simulink subsystem "Encoder_SubSystem"  (R2020b)
settings: Solver=VariableStepAuto  StartTime=0.0  StopTime=10.0  RelTol=1e-3
undefined symbols (not defined in the file or in its folder): n, sens, Ts
settings Model: Creator=umberto  LastModifiedBy=umberto

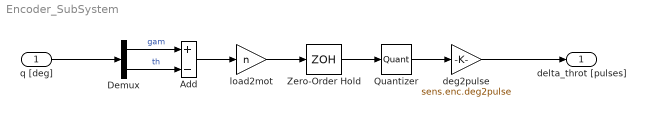
== system Encoder_SubSystem ==
  q [deg] : Inport
  Add : Sum  Inputs=+-
  Demux : Demux  Outputs=2
  Quantizer : Quantizer  QuantizationInterval=sens.enc.pulse2deg
  Zero-Order Hold : ZeroOrderHold  SampleTime=Ts
  deg2pulse : Gain  Gain=sens.enc.deg2pulse
  load2mot : Gain  Gain=n
  delta_throt [pulses] : Outport
  wires:
  q [deg]/1 -> Demux/1
  Demux/1 -> Add/1  "gam"
  Demux/2 -> Add/2  "th"
  Add/1 -> load2mot/1
  load2mot/1 -> Zero-Order Hold/1
  Zero-Order Hold/1 -> Quantizer/1
  Quantizer/1 -> deg2pulse/1
  deg2pulse/1 -> delta_throt [pulses]/1
